simulink model "spdobs"  (R2017a)
settings: Solver=FixedStepAuto  StartTime=0.0  StopTime=10.0  RelTol=1e-3  EnableMultiTasking=on
undefined symbols (not defined in the file): ctrl_lib, D, DiscIntNeverNeededParam, SPD_SM_K1, SPD_SM_K2
settings Model: Creator=uids8840  LastModifiedBy=root
settings SolverCC: AutoInsertRateTranBlk=on
settings OptimizationCC: DefaultParameterBehavior=Inlined  PassReuseOutputArgsAs=Individual arguments
settings DebuggingCC: ParameterTunabilityLossMsg=error
settings HardwareCC: ProdBitPerPointer=32  ProdBitPerSizeT=32  ProdBitPerPtrDiffT=32  ProdLargestAtomicInteger=Long  ProdLargestAtomicFloat=Double  ProdWordSize=32  ProdHWDeviceType=ARM Compatible->ARM Cortex
settings SFSimCC: MATLABDynamicMemAlloc=off
settings RTWCC: SystemTargetFile=ert.tlc  GenCodeOnly=on  PackageGeneratedCodeAndArtifacts=on  PackageName=spdobs  TemplateMakefile=ert_default_tmf  Description=Embedded Coder  GenerateReport=on  Toolchain=GNU gcc/g++ v4.4.x | gmake (64-bit Linux)  IncludeHyperlinkInReport=on  LaunchReport=on  GenerateTraceInfo=on  GenerateTraceReport=on  GenerateTraceReportSl=on  GenerateTraceReportSf=on  GenerateTraceReportEml=on
settings CodeAppCC: ForceParamTrailComments=on  IgnoreCustomStorageClasses=off  OperatorAnnotations=on  SimulinkDataObjDesc=on  SFDataObjDesc=on  MATLABFcnDesc=on  InsertBlockDesc=on  MATLABSourceComments=on
settings ERTTargetCC: TargetLangStandard=C99 (ISO)  SuppressErrorStatus=on  SupportAbsoluteTime=off  SupportNonFinite=off  SupportComplex=off  InlinedParameterPlacement=NonHierarchical  ERTCustomFileTemplate=example_file_process.tlc  GlobalDataDefinition=InSourceFile  GlobalDataReference=InSourceFile  ERTFilePackagingFormat=Compact

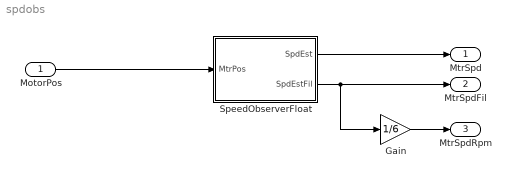
== system spdobs ==
  MotorPos : Inport  OutDataTypeStr=single
  Gain : Gain  Gain=1/6
  SpeedObserverFloat : Subsystem  SystemSampleTime=1e-4  RTWFcnName=SpdEst  RTWFileName=spdest
      settings: RTWFcnNameOpts=Use subsystem name  RTWFileNameOpts=Use subsystem name
  MtrSpd : Outport
  MtrSpdFil : Outport  Port=2
  MtrSpdRpm : Outport  Port=3
  wires:
  MotorPos/1 -> SpeedObserverFloat/1(MtrPos)
  SpeedObserverFloat/2(SpdEstFil) -> Gain/1, MtrSpdFil/1
  SpeedObserverFloat/1(SpdEst) -> MtrSpd/1
  Gain/1 -> MtrSpdRpm/1

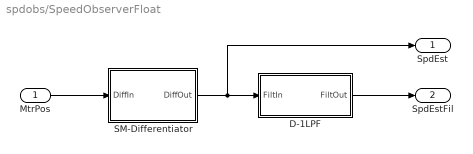
== system spdobs/SpeedObserverFloat ==
  MtrPos : Inport
  D-1LPF : Subsystem  AncestorBlock=ctrl_lib/D-1LPF  mask{tau=2.5e-3, ts=1/30e3}
      mask prompts: tau "Filter Constant [1/s]:"; ts "Execution Rate [s]:"
      mask DialogControl DescTextVar Prompt: Digital first order low pass filter.
  SM-Differentiator : Subsystem  TreatAsAtomicUnit=on  SystemSampleTime=1/30e3
  SpdEst : Outport
  SpdEstFil : Outport  Port=2
  wires:
  SM-Differentiator/1(DiffOut) -> SpdEst/1, D-1LPF/1(FiltIn)
  D-1LPF/1(FiltOut) -> SpdEstFil/1
  MtrPos/1 -> SM-Differentiator/1(DiffIn)

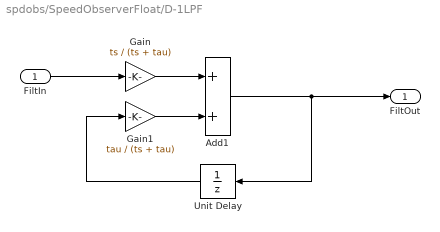
== system spdobs/SpeedObserverFloat/D-1LPF ==
  FiltIn : Inport
  Add1 : Sum
  Gain : Gain  Gain=ts / (ts + tau)  ParamDataTypeStr=Inherit: Inherit from 'Gain'  OutDataTypeStr=Inherit: Inherit via back propagation
  Gain1 : Gain  Gain=tau / (ts + tau)  ParamDataTypeStr=Inherit: Inherit from 'Gain'  OutDataTypeStr=Inherit: Inherit via back propagation
  Unit Delay : UnitDelay  SampleTime=-1
  FiltOut : Outport
  wires:
  FiltIn/1 -> Gain/1
  Unit Delay/1 -> Gain1/1
  Gain/1 -> Add1/1
  Add1/1 -> FiltOut/1, Unit Delay/1
  Gain1/1 -> Add1/2

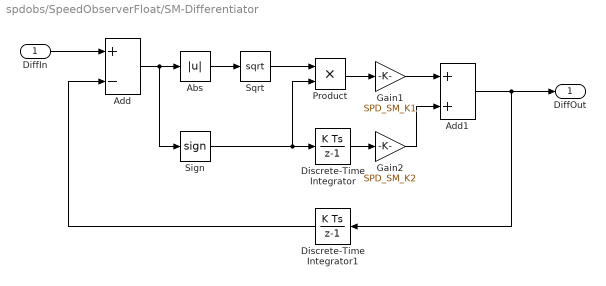
== system spdobs/SpeedObserverFloat/SM-Differentiator ==
  DiffIn : Inport
  Abs : Abs
  Add : Sum  Inputs=+-
  Add1 : Sum
  Discrete-Time Integrator : DiscreteIntegrator  InitialConditionSetting=State (most efficient)  SampleTime=-1  ICPrevOutput=DiscIntNeverNeededParam  ICPrevScaledInput=DiscIntNeverNeededParam
  Discrete-Time Integrator1 : DiscreteIntegrator  InitialConditionSetting=State (most efficient)  SampleTime=-1  ICPrevOutput=DiscIntNeverNeededParam  ICPrevScaledInput=DiscIntNeverNeededParam
  Gain1 : Gain  Gain=SPD_SM_K1
  Gain2 : Gain  Gain=SPD_SM_K2
  Product : Product
  Sign : Signum
  Sqrt : Sqrt  SaturateOnIntegerOverflow=on
  DiffOut : Outport
  wires:
  Add/1 -> Sign/1, Abs/1
  Gain2/1 -> Add1/2
  Product/1 -> Gain1/1
  Discrete-Time Integrator/1 -> Gain2/1
  Add1/1 -> DiffOut/1, Discrete-Time Integrator1/1
  Gain1/1 -> Add1/1
  Abs/1 -> Sqrt/1
  Sign/1 -> Product/2, Discrete-Time Integrator/1
  Discrete-Time Integrator1/1 -> Add/2
  Sqrt/1 -> Product/1
  DiffIn/1 -> Add/1
